simulink model "Cruise_Control_Simulink"  (R2022a)
settings: Solver=VariableStepAuto  StartTime=0.0  StopTime=Sim_Time  RelTol=1e-3
values from neighbouring files (symbols this model uses):
  A = h*w    (= 3.253845)    [Cruise_Control_Script.m]
  Cd = 0.4    [Cruise_Control_Script.m]
  Crr = 0.015    [Cruise_Control_Script.m]
  g = 9.81    [Cruise_Control_Script.m]
  kd = 100    [Cruise_Control_Script.m]
  ki = 18    [Cruise_Control_Script.m]
  kp = 350    [Cruise_Control_Script.m]
  M = 2300    [Cruise_Control_Script.m]
  rho = 1.293    [Cruise_Control_Script.m]
  v_actual = input('Enter current velocity in mph: ') / 2.237    [Cruise_Control_Script.m]
  v_desired = input('Enter desired velocity in mph: ') / 2.237    [Cruise_Control_Script.m]
  v_min = 30 / 2.237    (= 13.4108180599)    [Cruise_Control_Script.m]
settings Model: Creator=ao726  LastModifiedBy=ao726

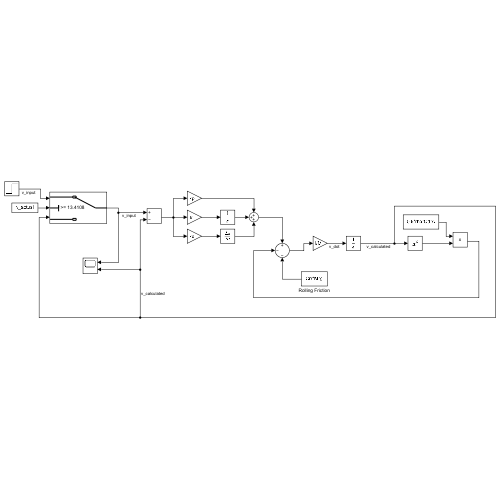
[thumbnail: Simulink's stored preview of the top-level diagram]
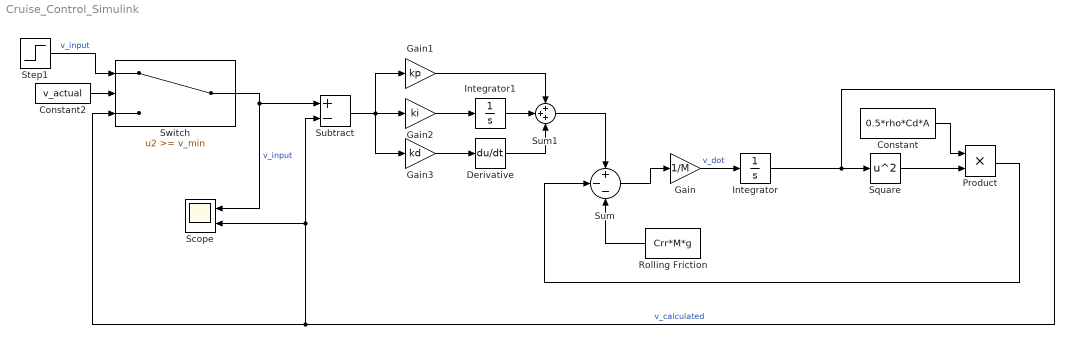
== system Cruise_Control_Simulink ==
  Constant : Constant  Value=0.5*rho*Cd*A
  Constant2 : Constant  Value=v_actual
  Derivative : Derivative
  Gain : Gain  Gain=1/M
  Gain1 : Gain  Gain=kp
  Gain2 : Gain  Gain=ki
  Gain3 : Gain  Gain=kd
  Integrator : Integrator  InitialCondition=v_actual
  Integrator1 : Integrator
  Product : Product
  Rolling Friction : Constant  Value=Crr*M*g
  Scope : Scope  NumInputPorts=2
  Square : Math  Operator=square
  Step1 : Step  Before=v_actual  After=v_desired  SampleTime=0
  Subtract : Sum  Inputs=+-
  Sum : Sum  Inputs=+--
  Sum1 : Sum  Inputs=+++
  Switch : Switch  Threshold=v_min  SaturateOnIntegerOverflow=off  InputSameDT=off
  wires:
  Gain/1 -> Integrator/1  "v_dot"
  Square/1 -> Product/2
  Constant/1 -> Product/1
  Product/1 -> Sum/2
  Rolling Friction/1 -> Sum/3
  Sum/1 -> Gain/1
  Gain2/1 -> Integrator1/1
  Gain3/1 -> Derivative/1
  Gain1/1 -> Sum1/1
  Integrator1/1 -> Sum1/2
  Derivative/1 -> Sum1/3
  Sum1/1 -> Sum/1
  Subtract/1 -> Gain3/1, Gain1/1, Gain2/1
  Switch/1 -> Subtract/1, Scope/1  "v_input"
  Step1/1 -> Switch/1  "v_input"
  Integrator/1 -> Square/1, Subtract/2, Scope/2, Switch/3  "v_calculated"
  Constant2/1 -> Switch/2
